simulink model "JULY"  (R2016b)
settings: Solver=VariableStepAuto  StartTime=0.0  StopTime=10  RelTol=1e-3
undefined symbols (not defined in the file): DiscIntNeverNeededParam
libraries: powerlib x8, powerlib_meascontrol x1
settings Model: Creator=sithuaung  LastModifiedBy=sithuaung

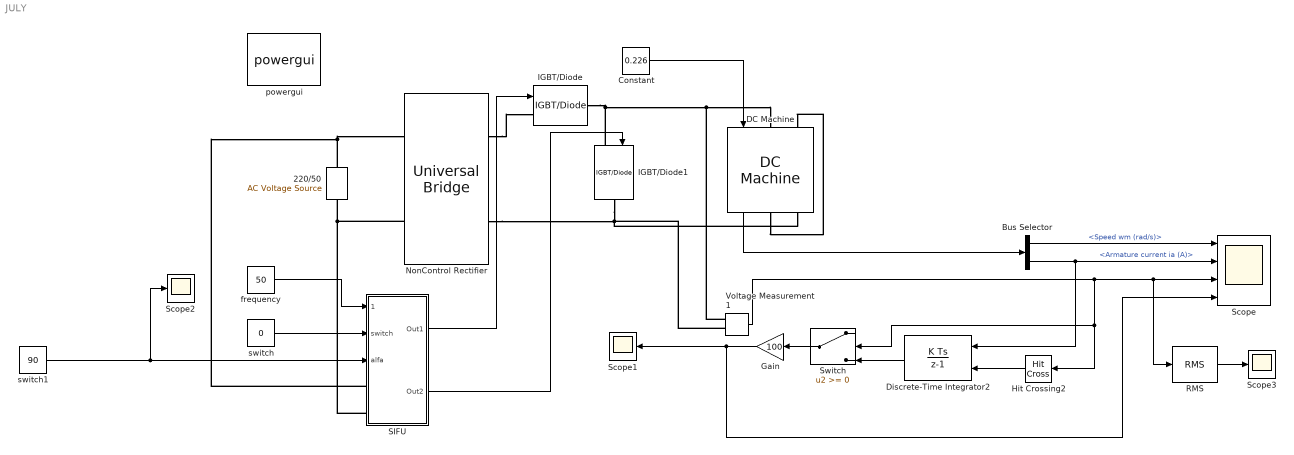
== system JULY ==
  220/50 : powerlib/Electrical Sources/AC Voltage Source  Amplitude=220*sqrt(2)  Phase=0  Frequency=50  SampleTime=0  Measurements=None  BusType=swing  Pref=10e3  Qref=0  Qmin=-inf  Qmax=+inf
  Bus Selector : BusSelector  OutputSignals=Speed wm (rad/s),Armature current ia (A)
  Constant : Constant  Value=0.226
  DC Machine : powerlib/Machines/DC Machine  PresetModel=No  MechanicalLoad=Torque TL  FieldType=Wound  ShowDetailedParameters=on  MeasurementBus=off  RLa="[ 7.061  0.058]"  RLf="[ 12.939  0.531]"  Laf=0.0098  MachineConstant=Torque constant (N.m/A)  Ke=1.8  Kt=1.8  J=0.21e-3  Bm=0  Tf=0  w0=1  Ifinit=-8.46539071434242e-022  TsPowergui=0  TsBlock=-1
      settings: AttributesFormatString=\n
  Discrete-Time Integrator2 : DiscreteIntegrator  gainval=1  ExternalReset=rising  SampleTime=2e-005  ICPrevOutput=DiscIntNeverNeededParam  ICPrevScaledInput=DiscIntNeverNeededParam
  Gain : Gain  Gain=100
  Hit Crossing2 : HitCross  HitCrossingDirection=rising  SampleTime=2e-005
  IGBT/Diode : powerlib/Power Electronics/IGBT//Diode  Ron=1e-3  Rs=1e5  Cs=inf  Measurements=off
  IGBT/Diode1 : powerlib/Power Electronics/IGBT//Diode  Ron=1e-3  Rs=1e5  Cs=inf  Measurements=off
  NonControl Rectifier : powerlib/Power Electronics/Universal Bridge  Arms=2  SnubberResistance=1e5  SnubberCapacitance=inf  Device=Diodes  Ron=1e-3  Lon=0  ForwardVoltages="[  0  0  ]"  ForwardVoltage=0  GTOparameters=[ 10e-6 , 20e-6 ]  IGBTparameters=[ 1e-6 , 2e-6 ]  Measurements=Device currents  Measurements_2=None  converterType=Rectifier
  RMS : powerlib_meascontrol/Measurements/RMS  TrueRMS=on  Freq=50  RMSInit=120  Ts=0
  SIFU : Subsystem
  Scope : Scope  NumInputPorts=4
  Scope1 : Scope
  Scope2 : Scope
  Scope3 : Scope
  Switch : Switch  ZeroCross=off
  Voltage Measurement1 : powerlib/Measurements/Voltage Measurement  PhasorSimulation=off  OutputType=Complex  PSBequivalent=0
  frequency : Constant  Value=50
  powergui : powerlib/powergui  Priority=1  SimulationMode=Continuous  SolverType=Tustin  SampleTime=50e-6  frequency=60  SPID=on  DisableSnubberDevices=off  DisableRonSwitches=off  DisableVfSwitches=on  SwTol=0  DisplayEquations=off  Interpol=off  ExternalGateDelay=off  methode=off  Ts=0  FunctionMessages=off  echomessages=off  HookPort=off  EnableUseOfTLC=off  x0status=blocks  frequencyindice=50  Pbase=100e6  ErrMax=1e-4  Iterations=50  UnitsV=kV  UnitsW=MW  buscounter=0  RestoreLinks=warning  ResistiveCurrentMeasurement=off  Frange=[0:2:500]  Ylog=off  Xlog=on  ShowGrid=off  save=off  variable=ZData  structure=rmsU  ZoomFFT=off  StartTime=0.0  cycles=1  DisplayStyle=1  fundamental=60  FreqAxis=off  MaxFrequency=1000  frequencyindicesteady=1  RmsSteady=1  display=off
  switch : Constant  Value=0
  switch1 : Constant  Value=90
  wires:
  DC Machine/1 -> Bus Selector/1
  Constant/1 -> DC Machine/1
  frequency/1 -> SIFU/1(frequency)
  switch/1 -> SIFU/2(switch)
  Bus Selector/2 -> Discrete-Time Integrator2/1, Scope/2  "<Armature current ia (A)>"
  SIFU/1(Out1) -> IGBT/Diode/1
  SIFU/2(Out2) -> IGBT/Diode1/1
  Hit Crossing2/1 -> Discrete-Time Integrator2/2
  Discrete-Time Integrator2/1 -> Switch/3
  Voltage Measurement1/1 -> Switch/2, Hit Crossing2/1, RMS/1, Scope/3
  Switch/1 -> Gain/1
  Gain/1 -> Scope1/1, Scope/4
  Bus Selector/1 -> Scope/1  "<Speed wm (rad/s)>"
  switch1/1 -> Scope2/1, SIFU/3(alfa)
  RMS/1 -> Scope3/1
  connections:
  NonControl Rectifier/RConn2 -- Voltage Measurement1/LConn2 -- DC Machine/RConn2 -- IGBT/Diode1/RConn1
  SIFU/LConn1 -- 220/50/RConn1 -- NonControl Rectifier/LConn1
  NonControl Rectifier/LConn2 -- 220/50/LConn1 -- SIFU/LConn2
  DC Machine/RConn1 -- DC Machine/LConn2
  NonControl Rectifier/RConn1 -- IGBT/Diode/LConn1
  IGBT/Diode/RConn1 -- Voltage Measurement1/LConn1 -- DC Machine/LConn1 -- IGBT/Diode1/LConn1

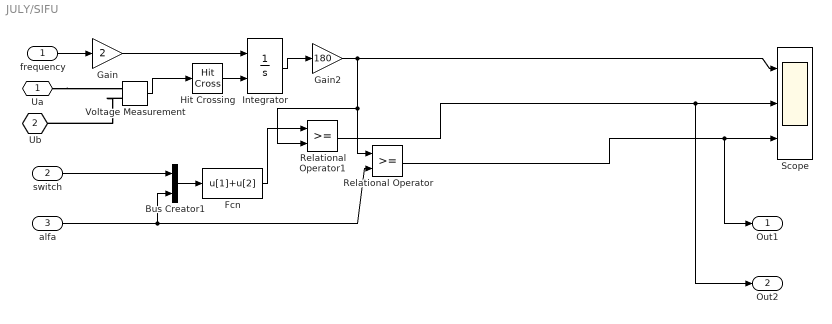
== system JULY/SIFU ==
  frequency : Inport
  switch : Inport  Port=2
  alfa : Inport  Port=3
  Bus Creator1 : BusCreator  Inputs=2
  Fcn : Fcn  Expr=u[1]+u[2]
  Gain : Gain  Gain=2
  Gain2 : Gain  Gain=180
  Hit Crossing : HitCross
  Integrator : Integrator  ExternalReset=either
  Relational Operator : RelationalOperator  OutDataTypeStr=boolean  RndMeth=Nearest
  Relational Operator1 : RelationalOperator  OutDataTypeStr=boolean  RndMeth=Nearest
  Scope : Scope  NumInputPorts=3
  Voltage Measurement : powerlib/Measurements/Voltage Measurement  PhasorSimulation=off  OutputType=Complex  PSBequivalent=0
  Ua : PMIOPort  Port=1  Side=Left
  Ub : PMIOPort  Port=2  Side=Left
  Out1 : Outport
  Out2 : Outport  Port=2
  wires:
  Integrator/1 -> Gain2/1
  Hit Crossing/1 -> Integrator/2
  Gain2/1 -> Scope/1, Relational Operator/1, Relational Operator1/2
  alfa/1 -> Bus Creator1/2, Relational Operator/2
  Bus Creator1/1 -> Fcn/1
  Fcn/1 -> Relational Operator1/1
  Relational Operator1/1 -> Out2/1, Scope/2
  Voltage Measurement/1 -> Hit Crossing/1
  frequency/1 -> Gain/1
  switch/1 -> Bus Creator1/1
  Gain/1 -> Integrator/1
  Relational Operator/1 -> Out1/1, Scope/3
  connections:
  Voltage Measurement/LConn2 -- Ub/RConn1
  Ua/RConn1 -- Voltage Measurement/LConn1
